simulink library "mylibrary"  (R2016b)
settings: Solver=VariableStepAuto  StartTime=0.0  StopTime=10.0  RelTol=1e-3
values from neighbouring files (symbols this model uses):
  bp_perio = bp_fft*2-3    (= 27)    [setup.m]
  Ewin = sum(wh.^2)/Nfft    [make_bias_plot_hann.m]    (also in setup.m = 1)
  N = M    [errAnalysis.m]    (also in make_bias_plot.m = 5; make_bias_plot_hann.m = 5; run_sim.m = 13; setup.m = 8)
  Nmax = 13    [setup.m]
  Ts = 1/fs    [create_test_vector.m]
libraries: xbsIndex_r4 x109, mylibrary x5, mylibrary_4printing x2
settings Model: Creator=susan  LastModifiedBy=292344
settings OptimizationCC: LifeSpan=inf
settings DebuggingCC: SFExecutionAtInitializationDiag=none

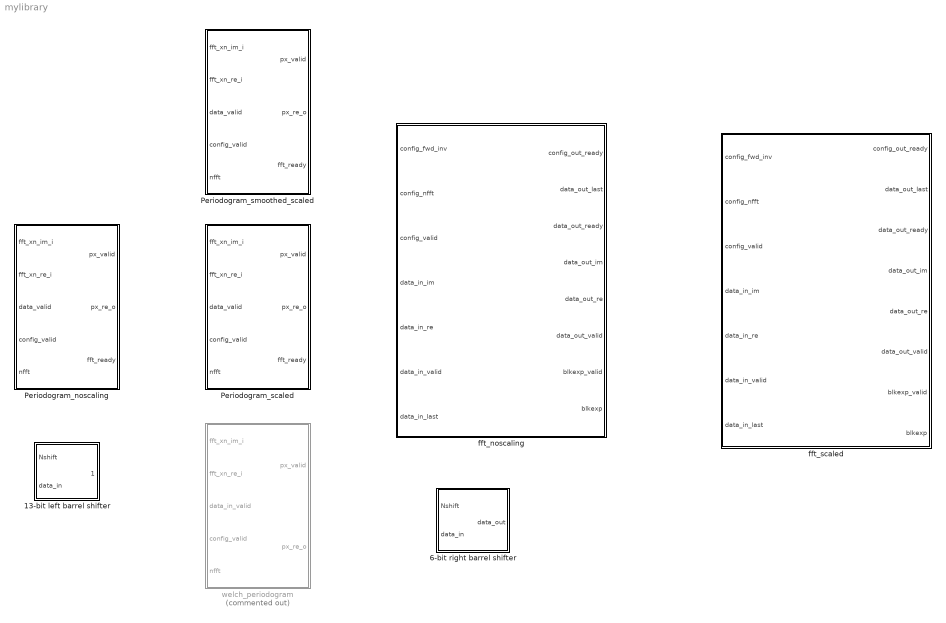
== system mylibrary ==
  13-bit left barrel shifter : Subsystem
  6-bit right barrel shifter : Subsystem
  Periodogram_noscaling : Subsystem
  Periodogram_scaled : Subsystem
  Periodogram_smoothed_scaled : Subsystem
  fft_noscaling : Subsystem
  fft_scaled : Subsystem
  welch_periodogram : Subsystem  Commented=on  AncestorBlock=mylibrary/smoothed_periodogram_scaled

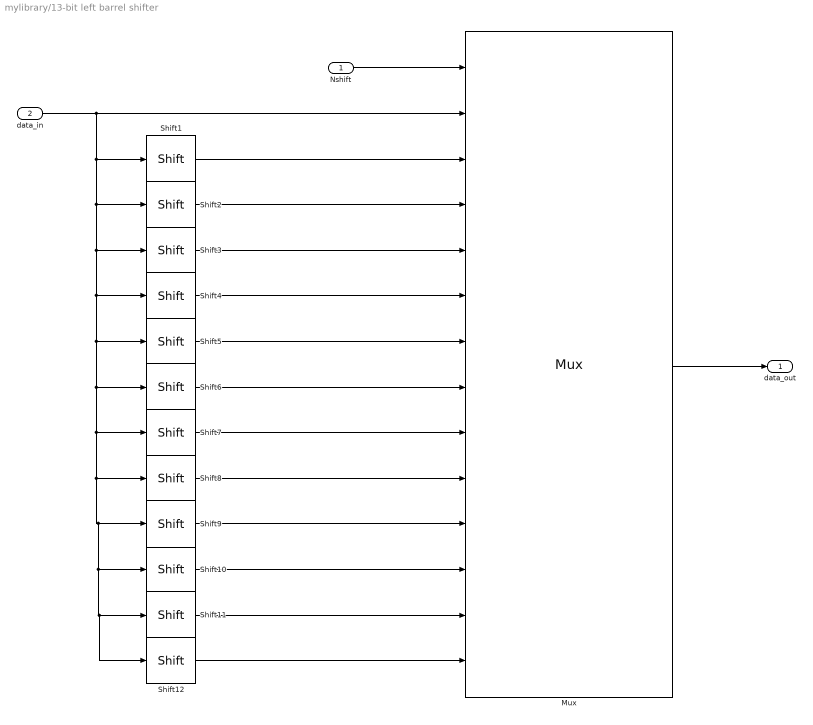
== system mylibrary/13-bit left barrel shifter ==
  Nshift : Inport
  data_in : Inport  Port=2
  Mux : xbsIndex_r4/Mux  inputs=13  en=off  latency=0  precision=Full  arith_type=Unsigned  n_bits=16  bin_pt=14  quantization=Truncate  overflow=Wrap  dbl_ovrd=off  block_type=mux
  Shift1 : xbsIndex_r4/Shift  shift_dir=Left  shift_bits=1  en=off  latency=0  precision=Full  arith_type="Signed  (2's comp)"  n_bits=16  bin_pt=14  quantization=Truncate  overflow=Wrap  dbl_ovrd=off  block_type=shift
  Shift10 : xbsIndex_r4/Shift  shift_dir=Left  shift_bits=10  en=off  latency=0  precision=Full  arith_type="Signed  (2's comp)"  n_bits=16  bin_pt=14  quantization=Truncate  overflow=Wrap  dbl_ovrd=off  block_type=shift
  Shift11 : xbsIndex_r4/Shift  shift_dir=Left  shift_bits=11  en=off  latency=0  precision=Full  arith_type="Signed  (2's comp)"  n_bits=16  bin_pt=14  quantization=Truncate  overflow=Wrap  dbl_ovrd=off  block_type=shift
  Shift12 : xbsIndex_r4/Shift  shift_dir=Left  shift_bits=12  en=off  latency=0  precision=Full  arith_type="Signed  (2's comp)"  n_bits=16  bin_pt=14  quantization=Truncate  overflow=Wrap  dbl_ovrd=off  block_type=shift
  Shift2 : xbsIndex_r4/Shift  shift_dir=Left  shift_bits=2  en=off  latency=0  precision=Full  arith_type="Signed  (2's comp)"  n_bits=16  bin_pt=14  quantization=Truncate  overflow=Wrap  dbl_ovrd=off  block_type=shift
  Shift3 : xbsIndex_r4/Shift  shift_dir=Left  shift_bits=3  en=off  latency=0  precision=Full  arith_type="Signed  (2's comp)"  n_bits=16  bin_pt=14  quantization=Truncate  overflow=Wrap  dbl_ovrd=off  block_type=shift
  Shift4 : xbsIndex_r4/Shift  shift_dir=Left  shift_bits=4  en=off  latency=0  precision=Full  arith_type="Signed  (2's comp)"  n_bits=16  bin_pt=14  quantization=Truncate  overflow=Wrap  dbl_ovrd=off  block_type=shift
  Shift5 : xbsIndex_r4/Shift  shift_dir=Left  shift_bits=5  en=off  latency=0  precision=Full  arith_type="Signed  (2's comp)"  n_bits=16  bin_pt=14  quantization=Truncate  overflow=Wrap  dbl_ovrd=off  block_type=shift
  Shift6 : xbsIndex_r4/Shift  shift_dir=Left  shift_bits=6  en=off  latency=0  precision=Full  arith_type="Signed  (2's comp)"  n_bits=16  bin_pt=14  quantization=Truncate  overflow=Wrap  dbl_ovrd=off  block_type=shift
  Shift7 : xbsIndex_r4/Shift  shift_dir=Left  shift_bits=7  en=off  latency=0  precision=Full  arith_type="Signed  (2's comp)"  n_bits=16  bin_pt=14  quantization=Truncate  overflow=Wrap  dbl_ovrd=off  block_type=shift
  Shift8 : xbsIndex_r4/Shift  shift_dir=Left  shift_bits=8  en=off  latency=0  precision=Full  arith_type="Signed  (2's comp)"  n_bits=16  bin_pt=14  quantization=Truncate  overflow=Wrap  dbl_ovrd=off  block_type=shift
  Shift9 : xbsIndex_r4/Shift  shift_dir=Left  shift_bits=9  en=off  latency=0  precision=Full  arith_type="Signed  (2's comp)"  n_bits=16  bin_pt=14  quantization=Truncate  overflow=Wrap  dbl_ovrd=off  block_type=shift
  data_out : Outport
  wires:
  Mux/1 -> data_out/1
  Nshift/1 -> Mux/1
  data_in/1 -> Shift12/1, Shift11/1, Shift10/1, Shift9/1, Shift8/1, Shift7/1, Shift6/1, Shift5/1, Shift4/1, Shift3/1, Shift2/1, Shift1/1, Mux/2
  Shift1/1 -> Mux/3
  Shift2/1 -> Mux/4
  Shift3/1 -> Mux/5
  Shift4/1 -> Mux/6
  Shift5/1 -> Mux/7
  Shift6/1 -> Mux/8
  Shift7/1 -> Mux/9
  Shift8/1 -> Mux/10
  Shift9/1 -> Mux/11
  Shift10/1 -> Mux/12
  Shift11/1 -> Mux/13
  Shift12/1 -> Mux/14

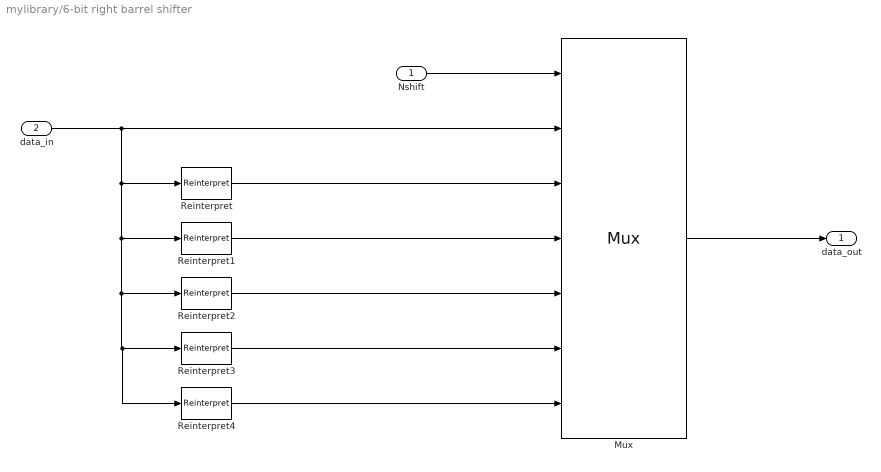
== system mylibrary/6-bit right barrel shifter ==
  Nshift : Inport
  data_in : Inport  Port=2
  Mux : xbsIndex_r4/Mux  inputs=6  en=off  latency=0  precision=Full  arith_type=Unsigned  n_bits=16  bin_pt=14  quantization=Truncate  overflow=Wrap  dbl_ovrd=off  block_type=mux
  Reinterpret : xbsIndex_r4/Reinterpret  force_arith_type=off  arith_type=Unsigned  force_bin_pt=on  bin_pt=bp_perio+1  block_type=reinterpret
  Reinterpret1 : xbsIndex_r4/Reinterpret  force_arith_type=off  arith_type=Unsigned  force_bin_pt=on  bin_pt=bp_perio+2  block_type=reinterpret
  Reinterpret2 : xbsIndex_r4/Reinterpret  force_arith_type=off  arith_type=Unsigned  force_bin_pt=on  bin_pt=bp_perio+3  block_type=reinterpret
  Reinterpret3 : xbsIndex_r4/Reinterpret  force_arith_type=off  arith_type=Unsigned  force_bin_pt=on  bin_pt=bp_perio+4  block_type=reinterpret
  Reinterpret4 : xbsIndex_r4/Reinterpret  force_arith_type=off  arith_type=Unsigned  force_bin_pt=on  bin_pt=bp_perio+5  block_type=reinterpret
  data_out : Outport
  wires:
  Nshift/1 -> Mux/1
  Mux/1 -> data_out/1
  Reinterpret/1 -> Mux/3
  Reinterpret1/1 -> Mux/4
  data_in/1 -> Reinterpret/1, Reinterpret4/1, Reinterpret3/1, Reinterpret2/1, Reinterpret1/1, Mux/2
  Reinterpret2/1 -> Mux/5
  Reinterpret3/1 -> Mux/6
  Reinterpret4/1 -> Mux/7

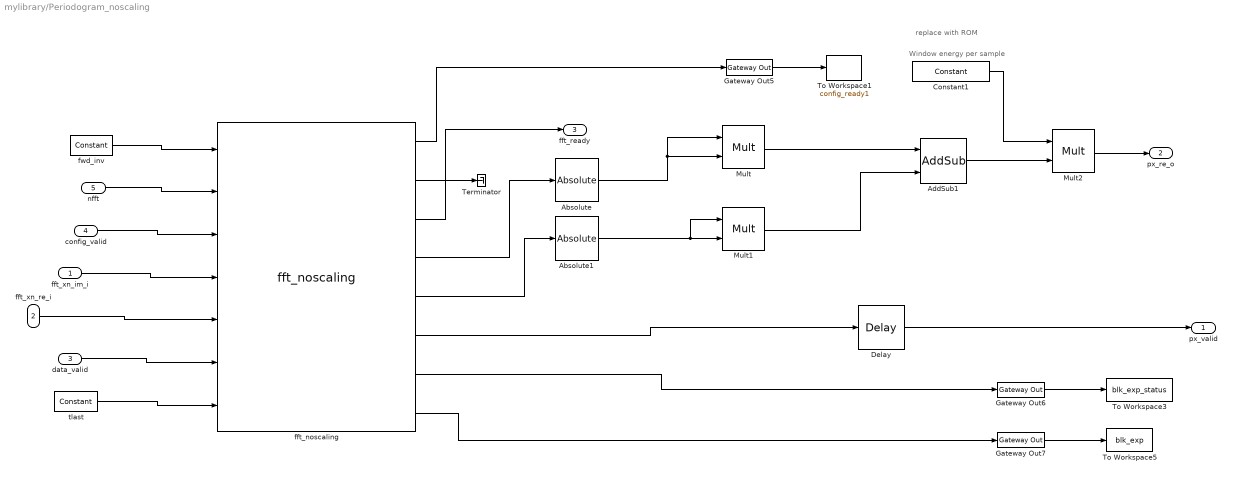
== system mylibrary/Periodogram_noscaling ==
  note: Window energy per sample
  note: replace with ROM
  fft_xn_im_i : Inport
  fft_xn_re_i : Inport  Port=2
  data_valid : Inport  Port=3
  config_valid : Inport  Port=4
  nfft : Inport  Port=5
  Absolute : xbsIndex_r4/Absolute  precision=User Defined  arith_type=Unsigned  n_bits=width_fft  bin_pt=bp_fft  quantization=Truncate  overflow=Wrap  en=off  latency=0  dbl_ovrd=off  block_type=abs
  Absolute1 : xbsIndex_r4/Absolute  precision=User Defined  arith_type=Unsigned  n_bits=width_fft  bin_pt=bp_fft  quantization=Truncate  overflow=Wrap  en=off  latency=0  dbl_ovrd=off  block_type=abs
  AddSub1 : xbsIndex_r4/AddSub  mode=Addition  use_carryin=off  use_carryout=off  en=off  latency=0  precision=Full  arith_type=Unsigned  n_bits=width_perio  bin_pt=bp_perio  quantization="Round  (unbiased: +/- Inf)"  overflow=Flag as error  use_behavioral_HDL=off  hw_selection=Fabric  pipelined=off  dbl_ovrd=off  block_type=addsub
  Constant1 : xbsIndex_r4/Constant  const=Ewin  gui_display_data_type=Fixed-point  arith_type=Unsigned  n_bits=32  bin_pt=20  preci_type=Single  exp_width=8  frac_width=24  explicit_period=on  period=1  equ=P=C  opselect=C  inp2=PCIN>>17  opr=+  inp1=P  carry=CIN  dbl_ovrd=off  block_type=constant
  Delay : xbsIndex_r4/Delay  rst=off  infoeditControl=Selection of Reset will increase slice count due to use of real FFs and instead of SRLs  en=off  latency=6  reg_retiming=off  dbl_ovrd=off  block_type=delay
      settings: infoedit=Hardware notes: A delay line is a chain, each link of which is an SRL16 or SRL32 followed by a flip-flop.
  Gateway Out5 : xbsIndex_r4/Gateway Out  inherit_from_input=off  hdl_port=on  rows=1  columns=1  UseAsDAC=off  DACChannel='1'  interface=None  automatic_assignment=on  address_offset=hex2dec('00')  intf_name=''  intf_description=''  timing_constraint=None  locs_specified=off  LOCs={}  io_standard={}  block_type=gatewayout
  Gateway Out6 : xbsIndex_r4/Gateway Out  inherit_from_input=off  hdl_port=on  rows=1  columns=1  UseAsDAC=off  DACChannel='1'  interface=None  automatic_assignment=on  address_offset=hex2dec('00')  intf_name=''  intf_description=''  timing_constraint=None  locs_specified=off  LOCs={}  io_standard={}  block_type=gatewayout
  Gateway Out7 : xbsIndex_r4/Gateway Out  inherit_from_input=off  hdl_port=on  rows=1  columns=1  UseAsDAC=off  DACChannel='1'  interface=None  automatic_assignment=on  address_offset=hex2dec('00')  intf_name=''  intf_description=''  timing_constraint=None  locs_specified=off  LOCs={}  io_standard={}  block_type=gatewayout
  Mult : xbsIndex_r4/Mult  precision=Full  arith_type=Unsigned  n_bits=width_perio  bin_pt=bp_perio  quantization="Round  (unbiased: +/- Inf)"  overflow=Wrap  en=off  latency=3  use_behavioral_HDL=off  opt=Speed  use_embedded=on  optimum_pipeline=off  pipeline=on  dbl_ovrd=off  use_rpm=on  placement_style=Triangular  block_type=mult
  Mult1 : xbsIndex_r4/Mult  precision=Full  arith_type=Unsigned  n_bits=width_perio  bin_pt=bp_perio  quantization="Round  (unbiased: +/- Inf)"  overflow=Wrap  en=off  latency=3  use_behavioral_HDL=off  opt=Speed  use_embedded=on  optimum_pipeline=off  pipeline=on  dbl_ovrd=off  use_rpm=on  placement_style=Triangular  block_type=mult
  Mult2 : xbsIndex_r4/Mult  precision=User Defined  arith_type=Unsigned  n_bits=width_perio  bin_pt=bp_perio  quantization="Round  (unbiased: +/- Inf)"  overflow=Flag as error  en=off  latency=3  use_behavioral_HDL=off  opt=Speed  use_embedded=on  optimum_pipeline=off  pipeline=on  dbl_ovrd=off  use_rpm=on  placement_style=Triangular  block_type=mult
  Terminator : Terminator
  To Workspace1 : ToWorkspace  VariableName=config_ready1  SaveFormat=Timeseries  SampleTime=-1
  To Workspace3 : ToWorkspace  VariableName=blk_exp_status  SaveFormat=Timeseries  SampleTime=-1
  To Workspace5 : ToWorkspace  VariableName=blk_exp  SaveFormat=Timeseries  SampleTime=-1
  fft_noscaling : mylibrary/fft_noscaling
  fwd_inv : xbsIndex_r4/Constant  const=1.0  gui_display_data_type=Fixed-point  arith_type=Unsigned  n_bits=1  bin_pt=0  preci_type=Single  exp_width=8  frac_width=24  explicit_period=off  period=1  equ=P=C  opselect=C  inp2=PCIN>>17  opr=+  inp1=P  carry=CIN  dbl_ovrd=off  block_type=constant
  tlast : xbsIndex_r4/Constant  const=1.0  gui_display_data_type=Boolean  arith_type=Boolean  n_bits=16  bin_pt=14  preci_type=Single  exp_width=8  frac_width=24  explicit_period=off  period=1  equ=P=C  opselect=C  inp2=PCIN>>17  opr=+  inp1=P  carry=CIN  dbl_ovrd=off  block_type=constant
  px_valid : Outport
  px_re_o : Outport  Port=2
  fft_ready : Outport  Port=3
  wires:
  Delay/1 -> px_valid/1
  Mult/1 -> AddSub1/1
  Mult1/1 -> AddSub1/2
  Gateway Out5/1 -> To Workspace1/1
  Absolute/1 -> Mult/2, Mult/1
  Absolute1/1 -> Mult1/1, Mult1/2
  AddSub1/1 -> Mult2/2
  Mult2/1 -> px_re_o/1
  Constant1/1 -> Mult2/1
  fft_noscaling/5 -> Absolute1/1
  fft_noscaling/6 -> Delay/1
  fft_noscaling/4 -> Absolute/1
  fwd_inv/1 -> fft_noscaling/1
  nfft/1 -> fft_noscaling/2
  config_valid/1 -> fft_noscaling/3
  fft_xn_im_i/1 -> fft_noscaling/4
  fft_xn_re_i/1 -> fft_noscaling/5
  data_valid/1 -> fft_noscaling/6
  tlast/1 -> fft_noscaling/7
  fft_noscaling/1 -> Gateway Out5/1
  fft_noscaling/3 -> fft_ready/1
  Gateway Out6/1 -> To Workspace3/1
  Gateway Out7/1 -> To Workspace5/1
  fft_noscaling/7 -> Gateway Out6/1
  fft_noscaling/8 -> Gateway Out7/1
  fft_noscaling/2 -> Terminator/1

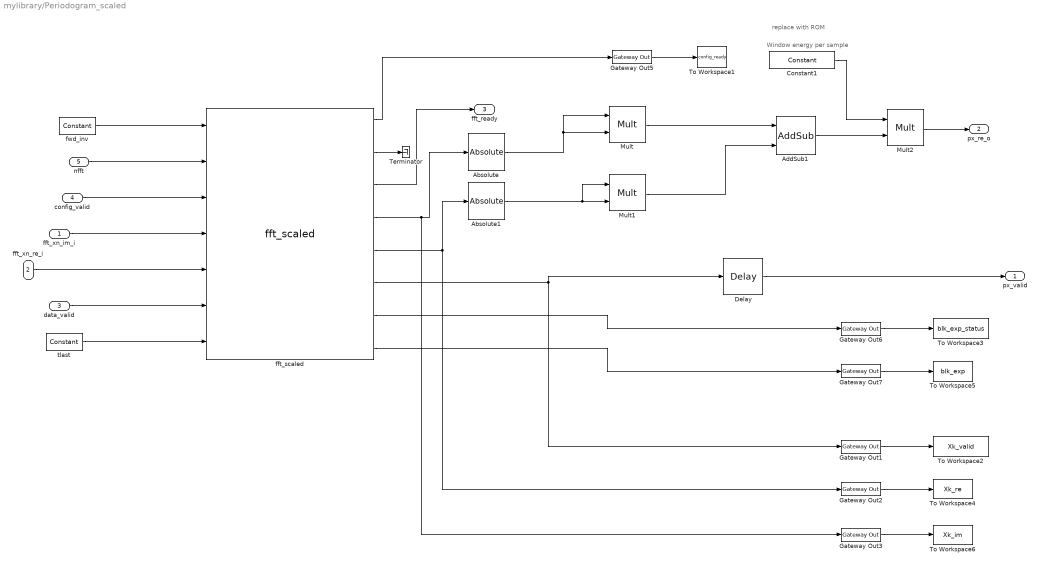
== system mylibrary/Periodogram_scaled ==
  note: replace with ROM
  note: Window energy per sample
  fft_xn_im_i : Inport
  fft_xn_re_i : Inport  Port=2
  data_valid : Inport  Port=3
  config_valid : Inport  Port=4
  nfft : Inport  Port=5
  Absolute : xbsIndex_r4/Absolute  precision=User Defined  arith_type=Unsigned  n_bits=width_fft  bin_pt=bp_fft  quantization=Truncate  overflow=Wrap  en=off  latency=0  dbl_ovrd=off  block_type=abs
  Absolute1 : xbsIndex_r4/Absolute  precision=User Defined  arith_type=Unsigned  n_bits=width_fft  bin_pt=bp_fft  quantization=Truncate  overflow=Wrap  en=off  latency=0  dbl_ovrd=off  block_type=abs
  AddSub1 : xbsIndex_r4/AddSub  mode=Addition  use_carryin=off  use_carryout=off  en=off  latency=0  precision=Full  arith_type=Unsigned  n_bits=width_perio  bin_pt=bp_perio  quantization="Round  (unbiased: +/- Inf)"  overflow=Flag as error  use_behavioral_HDL=off  hw_selection=Fabric  pipelined=off  dbl_ovrd=off  block_type=addsub
  Constant1 : xbsIndex_r4/Constant  const=Ewin  gui_display_data_type=Fixed-point  arith_type=Unsigned  n_bits=32  bin_pt=20  preci_type=Single  exp_width=8  frac_width=24  explicit_period=on  period=1  equ=P=C  opselect=C  inp2=PCIN>>17  opr=+  inp1=P  carry=CIN  dbl_ovrd=off  block_type=constant
  Delay : xbsIndex_r4/Delay  rst=off  infoeditControl=Selection of Reset will increase slice count due to use of real FFs and instead of SRLs  en=off  latency=6  reg_retiming=off  dbl_ovrd=off  block_type=delay
      settings: infoedit=Hardware notes: A delay line is a chain, each link of which is an SRL16 or SRL32 followed by a flip-flop.
  Gateway Out{1..3,5..7} (6 alike) : xbsIndex_r4/Gateway Out  inherit_from_input=off  hdl_port=on  rows=1  columns=1  UseAsDAC=off  DACChannel='1'  interface=None  automatic_assignment=on  address_offset=hex2dec('00')  intf_name=''  intf_description=''  timing_constraint=None  locs_specified=off  LOCs={}  io_standard={}  block_type=gatewayout
  Mult : xbsIndex_r4/Mult  precision=Full  arith_type=Unsigned  n_bits=width_perio  bin_pt=bp_perio  quantization="Round  (unbiased: +/- Inf)"  overflow=Wrap  en=off  latency=3  use_behavioral_HDL=off  opt=Speed  use_embedded=on  optimum_pipeline=off  pipeline=on  dbl_ovrd=off  use_rpm=on  placement_style=Triangular  block_type=mult
  Mult1 : xbsIndex_r4/Mult  precision=Full  arith_type=Unsigned  n_bits=width_perio  bin_pt=bp_perio  quantization="Round  (unbiased: +/- Inf)"  overflow=Wrap  en=off  latency=3  use_behavioral_HDL=off  opt=Speed  use_embedded=on  optimum_pipeline=off  pipeline=on  dbl_ovrd=off  use_rpm=on  placement_style=Triangular  block_type=mult
  Mult2 : xbsIndex_r4/Mult  precision=User Defined  arith_type=Unsigned  n_bits=width_perio  bin_pt=bp_perio  quantization="Round  (unbiased: +/- Inf)"  overflow=Flag as error  en=off  latency=3  use_behavioral_HDL=off  opt=Speed  use_embedded=on  optimum_pipeline=off  pipeline=on  dbl_ovrd=off  use_rpm=on  placement_style=Triangular  block_type=mult
  Terminator : Terminator
  To Workspace1 : ToWorkspace  VariableName=config_ready  SaveFormat=Timeseries  SampleTime=-1
  To Workspace2 : ToWorkspace  VariableName=Xk_valid  SaveFormat=Timeseries  SampleTime=-1
  To Workspace3 : ToWorkspace  VariableName=blk_exp_status  SaveFormat=Timeseries  SampleTime=-1
  To Workspace4 : ToWorkspace  VariableName=Xk_re  SaveFormat=Timeseries  SampleTime=-1
  To Workspace5 : ToWorkspace  VariableName=blk_exp  SaveFormat=Timeseries  SampleTime=-1
  To Workspace6 : ToWorkspace  VariableName=Xk_im  SaveFormat=Timeseries  SampleTime=-1
  fft_scaled : mylibrary/fft_scaled
  fwd_inv : xbsIndex_r4/Constant  const=1.0  gui_display_data_type=Fixed-point  arith_type=Unsigned  n_bits=1  bin_pt=0  preci_type=Single  exp_width=8  frac_width=24  explicit_period=off  period=1  equ=P=C  opselect=C  inp2=PCIN>>17  opr=+  inp1=P  carry=CIN  dbl_ovrd=off  block_type=constant
  tlast : xbsIndex_r4/Constant  const=1.0  gui_display_data_type=Boolean  arith_type=Boolean  n_bits=16  bin_pt=14  preci_type=Single  exp_width=8  frac_width=24  explicit_period=off  period=1  equ=P=C  opselect=C  inp2=PCIN>>17  opr=+  inp1=P  carry=CIN  dbl_ovrd=off  block_type=constant
  px_valid : Outport
  px_re_o : Outport  Port=2
  fft_ready : Outport  Port=3
  wires:
  fft_scaled/2 -> Terminator/1
  fft_scaled/8 -> Gateway Out7/1
  fft_scaled/7 -> Gateway Out6/1
  Gateway Out7/1 -> To Workspace5/1
  Gateway Out6/1 -> To Workspace3/1
  fft_scaled/3 -> fft_ready/1
  fft_scaled/1 -> Gateway Out5/1
  tlast/1 -> fft_scaled/7
  data_valid/1 -> fft_scaled/6
  fft_xn_re_i/1 -> fft_scaled/5
  fft_xn_im_i/1 -> fft_scaled/4
  config_valid/1 -> fft_scaled/3
  nfft/1 -> fft_scaled/2
  fwd_inv/1 -> fft_scaled/1
  fft_scaled/4 -> Gateway Out3/1, Absolute/1
  fft_scaled/6 -> Gateway Out1/1, Delay/1
  fft_scaled/5 -> Gateway Out2/1, Absolute1/1
  Constant1/1 -> Mult2/1
  Mult2/1 -> px_re_o/1
  AddSub1/1 -> Mult2/2
  Absolute1/1 -> Mult1/2, Mult1/1
  Absolute/1 -> Mult/1, Mult/2
  Gateway Out5/1 -> To Workspace1/1
  Mult1/1 -> AddSub1/2
  Mult/1 -> AddSub1/1
  Delay/1 -> px_valid/1
  Gateway Out2/1 -> To Workspace4/1
  Gateway Out1/1 -> To Workspace2/1
  Gateway Out3/1 -> To Workspace6/1

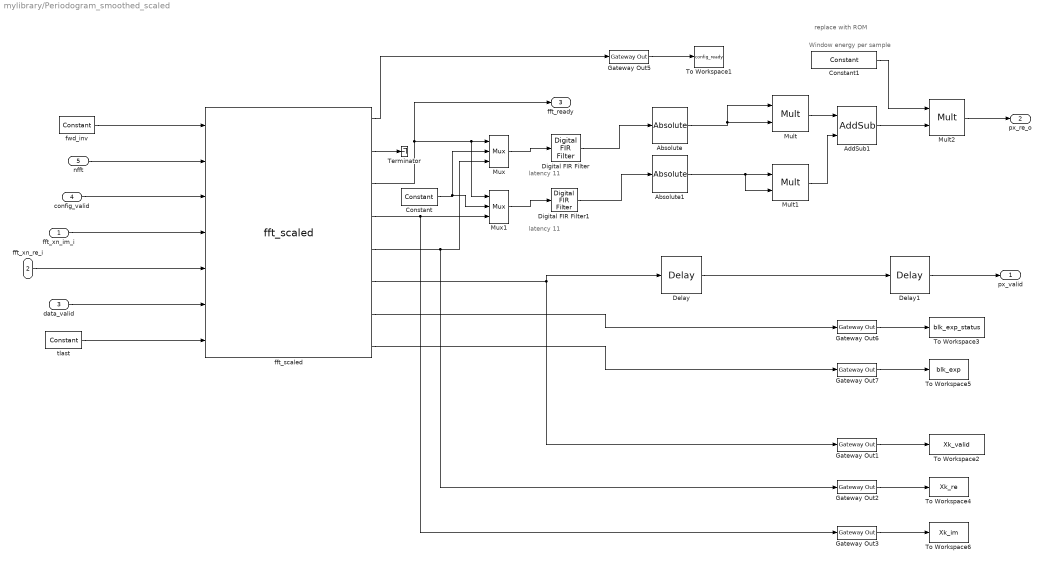
== system mylibrary/Periodogram_smoothed_scaled ==
  note: latency 11
  note: replace with ROM
  note: Window energy per sample
  note: latency 11
  fft_xn_im_i : Inport
  fft_xn_re_i : Inport  Port=2
  data_valid : Inport  Port=3
  config_valid : Inport  Port=4
  nfft : Inport  Port=5
  Absolute : xbsIndex_r4/Absolute  precision=User Defined  arith_type=Unsigned  n_bits=width_fft  bin_pt=bp_fft  quantization=Truncate  overflow=Wrap  en=off  latency=0  dbl_ovrd=off  block_type=abs
  Absolute1 : xbsIndex_r4/Absolute  precision=User Defined  arith_type=Unsigned  n_bits=width_fft  bin_pt=bp_fft  quantization=Truncate  overflow=Wrap  en=off  latency=0  dbl_ovrd=off  block_type=abs
  AddSub1 : xbsIndex_r4/AddSub  mode=Addition  use_carryin=off  use_carryout=off  en=off  latency=0  precision=Full  arith_type=Unsigned  n_bits=width_perio  bin_pt=bp_perio  quantization="Round  (unbiased: +/- Inf)"  overflow=Flag as error  use_behavioral_HDL=off  hw_selection=Fabric  pipelined=off  dbl_ovrd=off  block_type=addsub
  Constant : xbsIndex_r4/Constant  const=0  gui_display_data_type=Fixed-point  arith_type=Signed (2's comp)  n_bits=16  bin_pt=14  preci_type=Single  exp_width=8  frac_width=24  explicit_period=off  period=1  equ=P=C  opselect=C  inp2=PCIN>>17  opr=+  inp1=P  carry=CIN  dbl_ovrd=off  block_type=constant
  Constant1 : xbsIndex_r4/Constant  const=Ewin  gui_display_data_type=Fixed-point  arith_type=Unsigned  n_bits=32  bin_pt=20  preci_type=Single  exp_width=8  frac_width=24  explicit_period=on  period=1  equ=P=C  opselect=C  inp2=PCIN>>17  opr=+  inp1=P  carry=CIN  dbl_ovrd=off  block_type=constant
  Delay : xbsIndex_r4/Delay  rst=off  infoeditControl=Selection of Reset will increase slice count due to use of real FFs and instead of SRLs  en=off  latency=3  reg_retiming=off  dbl_ovrd=off  block_type=delay
  Delay1 : xbsIndex_r4/Delay  rst=off  infoeditControl=Selection of Reset will increase slice count due to use of real FFs and instead of SRLs  en=off  latency=14  reg_retiming=off  dbl_ovrd=off  block_type=delay
  Digital FIR Filter : xbsIndex_r4/Digital FIR Filter  coeff_source=off  coefficientvector=[-.25,0.5,-0.25]  coeff_calulate=on  coefficient_width=2  coefficient_fractional_bits=1  interpolation_filter_rate=1  decimation_filter_rate=1  fda_coefficientvector=[-0.0024 -0.0042 0.0095 0.0200 -0.0380 -0.0696 0.1374 0.4472 0.4472 0.1374 -0.0696 -0.0380 0.0200 0.0095 -0.0042 -0.0024]  simulation_type=fast_sim  simulation_model=sysgen:fir_macro  block_type=fir_macro
  Digital FIR Filter1 : xbsIndex_r4/Digital FIR Filter  coeff_source=off  coefficientvector=[-.25,0.5,-0.25]  coeff_calulate=on  coefficient_width=2  coefficient_fractional_bits=1  interpolation_filter_rate=1  decimation_filter_rate=1  fda_coefficientvector=[-0.0024 -0.0042 0.0095 0.0200 -0.0380 -0.0696 0.1374 0.4472 0.4472 0.1374 -0.0696 -0.0380 0.0200 0.0095 -0.0042 -0.0024]  simulation_type=fast_sim  simulation_model=sysgen:fir_macro  block_type=fir_macro
  Gateway Out{1..3,5..7} (6 alike) : xbsIndex_r4/Gateway Out  inherit_from_input=off  hdl_port=on  rows=1  columns=1  UseAsDAC=off  DACChannel='1'  interface=None  automatic_assignment=on  address_offset=hex2dec('00')  intf_name=''  intf_description=''  timing_constraint=None  locs_specified=off  LOCs={}  io_standard={}  block_type=gatewayout
  Mult : xbsIndex_r4/Mult  precision=Full  arith_type=Unsigned  n_bits=width_perio  bin_pt=bp_perio  quantization="Round  (unbiased: +/- Inf)"  overflow=Wrap  en=off  latency=3  use_behavioral_HDL=off  opt=Speed  use_embedded=on  optimum_pipeline=off  pipeline=on  dbl_ovrd=off  use_rpm=on  placement_style=Triangular  block_type=mult
  Mult1 : xbsIndex_r4/Mult  precision=Full  arith_type=Unsigned  n_bits=width_perio  bin_pt=bp_perio  quantization="Round  (unbiased: +/- Inf)"  overflow=Wrap  en=off  latency=3  use_behavioral_HDL=off  opt=Speed  use_embedded=on  optimum_pipeline=off  pipeline=on  dbl_ovrd=off  use_rpm=on  placement_style=Triangular  block_type=mult
  Mult2 : xbsIndex_r4/Mult  precision=User Defined  arith_type=Unsigned  n_bits=width_perio  bin_pt=bp_perio  quantization="Round  (unbiased: +/- Inf)"  overflow=Flag as error  en=off  latency=3  use_behavioral_HDL=off  opt=Speed  use_embedded=on  optimum_pipeline=off  pipeline=on  dbl_ovrd=off  use_rpm=on  placement_style=Triangular  block_type=mult
  Mux : xbsIndex_r4/Mux  inputs=2  en=off  latency=0  precision=Full  arith_type=Unsigned  n_bits=16  bin_pt=14  quantization=Truncate  overflow=Wrap  dbl_ovrd=off  block_type=mux
  Mux1 : xbsIndex_r4/Mux  inputs=2  en=off  latency=0  precision=Full  arith_type=Unsigned  n_bits=16  bin_pt=14  quantization=Truncate  overflow=Wrap  dbl_ovrd=off  block_type=mux
  Terminator : Terminator
  To Workspace1 : ToWorkspace  VariableName=config_ready  SaveFormat=Timeseries  SampleTime=-1
  To Workspace2 : ToWorkspace  VariableName=Xk_valid  SaveFormat=Timeseries  SampleTime=-1
  To Workspace3 : ToWorkspace  VariableName=blk_exp_status  SaveFormat=Timeseries  SampleTime=-1
  To Workspace4 : ToWorkspace  VariableName=Xk_re  SaveFormat=Timeseries  SampleTime=-1
  To Workspace5 : ToWorkspace  VariableName=blk_exp  SaveFormat=Timeseries  SampleTime=-1
  To Workspace6 : ToWorkspace  VariableName=Xk_im  SaveFormat=Timeseries  SampleTime=-1
  fft_scaled : mylibrary/fft_scaled
  fwd_inv : xbsIndex_r4/Constant  const=1.0  gui_display_data_type=Fixed-point  arith_type=Unsigned  n_bits=1  bin_pt=0  preci_type=Single  exp_width=8  frac_width=24  explicit_period=off  period=1  equ=P=C  opselect=C  inp2=PCIN>>17  opr=+  inp1=P  carry=CIN  dbl_ovrd=off  block_type=constant
  tlast : xbsIndex_r4/Constant  const=1.0  gui_display_data_type=Boolean  arith_type=Boolean  n_bits=16  bin_pt=14  preci_type=Single  exp_width=8  frac_width=24  explicit_period=off  period=1  equ=P=C  opselect=C  inp2=PCIN>>17  opr=+  inp1=P  carry=CIN  dbl_ovrd=off  block_type=constant
  px_valid : Outport
  px_re_o : Outport  Port=2
  fft_ready : Outport  Port=3
  wires:
  fft_scaled/2 -> Terminator/1
  fft_scaled/8 -> Gateway Out7/1
  fft_scaled/7 -> Gateway Out6/1
  Gateway Out7/1 -> To Workspace5/1
  Gateway Out6/1 -> To Workspace3/1
  fft_scaled/3 -> Mux1/1, Mux/1, fft_ready/1
  fft_scaled/1 -> Gateway Out5/1
  tlast/1 -> fft_scaled/7
  data_valid/1 -> fft_scaled/6
  fft_xn_re_i/1 -> fft_scaled/5
  fft_xn_im_i/1 -> fft_scaled/4
  config_valid/1 -> fft_scaled/3
  nfft/1 -> fft_scaled/2
  fwd_inv/1 -> fft_scaled/1
  fft_scaled/4 -> Mux1/3, Gateway Out3/1
  fft_scaled/6 -> Gateway Out1/1, Delay/1
  fft_scaled/5 -> Mux/3, Gateway Out2/1
  Constant1/1 -> Mult2/1
  Mult2/1 -> px_re_o/1
  Absolute1/1 -> Mult1/2, Mult1/1
  Absolute/1 -> Mult/1, Mult/2
  Gateway Out5/1 -> To Workspace1/1
  Mult1/1 -> AddSub1/2
  Mult/1 -> AddSub1/1
  Delay/1 -> Delay1/1
  Gateway Out2/1 -> To Workspace4/1
  Gateway Out1/1 -> To Workspace2/1
  Gateway Out3/1 -> To Workspace6/1
  Delay1/1 -> px_valid/1
  Mux/1 -> Digital FIR Filter/1
  AddSub1/1 -> Mult2/2
  Digital FIR Filter/1 -> Absolute/1
  Mux1/1 -> Digital FIR Filter1/1
  Digital FIR Filter1/1 -> Absolute1/1
  Constant/1 -> Mux1/2, Mux/2

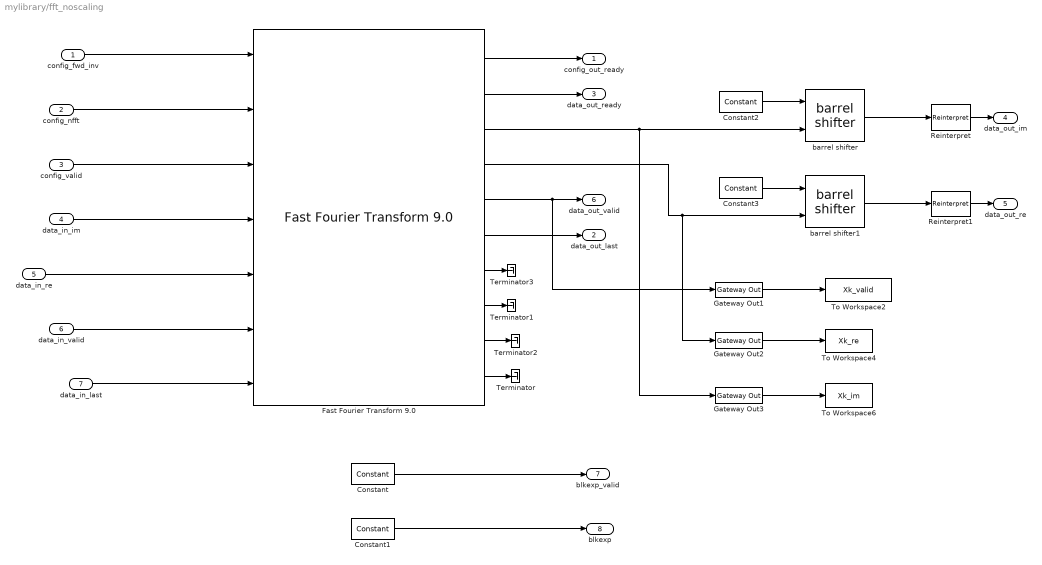
== system mylibrary/fft_noscaling ==
  config_fwd_inv : Inport
  config_nfft : Inport  Port=2
  config_valid : Inport  Port=3
  data_in_im : Inport  Port=4
  data_in_re : Inport  Port=5
  data_in_valid : Inport  Port=6
  data_in_last : Inport  Port=7
  Constant : xbsIndex_r4/Constant  const=1.0  gui_display_data_type=Boolean  arith_type=Boolean  n_bits=16  bin_pt=14  preci_type=Single  exp_width=8  frac_width=24  explicit_period=off  period=1  equ=P=C  opselect=C  inp2=PCIN>>17  opr=+  inp1=P  carry=CIN  dbl_ovrd=off  block_type=constant
  Constant1 : xbsIndex_r4/Constant  const=N  gui_display_data_type=Fixed-point  arith_type=Unsigned  n_bits=5  bin_pt=0  preci_type=Single  exp_width=8  frac_width=24  explicit_period=off  period=1  equ=P=C  opselect=C  inp2=PCIN>>17  opr=+  inp1=P  carry=CIN  dbl_ovrd=off  block_type=constant
  Constant2 : xbsIndex_r4/Constant  const=Nmax-N  gui_display_data_type=Fixed-point  arith_type=Unsigned  n_bits=4  bin_pt=0  preci_type=Single  exp_width=8  frac_width=24  explicit_period=off  period=1  equ=P=C  opselect=C  inp2=PCIN>>17  opr=+  inp1=P  carry=CIN  dbl_ovrd=off  block_type=constant
  Constant3 : xbsIndex_r4/Constant  const=Nmax-N  gui_display_data_type=Fixed-point  arith_type=Unsigned  n_bits=4  bin_pt=0  preci_type=Single  exp_width=8  frac_width=24  explicit_period=off  period=1  equ=P=C  opselect=C  inp2=PCIN>>17  opr=+  inp1=P  carry=CIN  dbl_ovrd=off  block_type=constant
  "Fast Fourier Transform 9.0 " : xbsIndex_r4/Fast Fourier Transform 9.0   transform_length=8192  target_clock_frequency=ceil(1/(Ts*1e6))  target_data_throughput=50  implementation_options=pipelined_streaming_io  run_time_configurable_transform_length=on  phase_factor_width=13  scaling_options=unscaled  rounding_modes=convergent_rounding  aclken=off  aresetn=off  output_ordering=natural_order  cyclic_prefix_insertion=off  throttle_scheme=realtime  xk_index=off  ovflo=off  trim_axipin_name=on  memory_options_data=block_ram  memory_options_phase_factors=block_ram  number_of_stages_using_block_ram_for_data_and_phase_factors=4  memory_options_reorder=block_ram  memory_options_hybrid=off  complex_mult_type=use_mults_performance  butterfly_type=use_luts  simulation_type=hybrid_sim  simulation_model=sysgen:xfftv9_cmodel  data_path_portlist={ 's_axis_data_tdata', 'm_axis_data_tdata', 'm_axis_status_tdata', 'event_fft_overflow' }  channels=1  input_ordering=natural_order  input_width=16  ip_name=Fast Fourier Transform  ip_version=9.0  dsptool_ready=true  ipcore_usecache=true  ipcore_useipmodelcache=true  wrapper_available=true  port_translation_map={ 'aclken' => 'en', 'aresetn' => 'rst'}  data_format=fixed_point  block_type=xfft_v9_0
  Gateway Out1 : xbsIndex_r4/Gateway Out  inherit_from_input=off  hdl_port=on  rows=1  columns=1  UseAsDAC=off  DACChannel='1'  interface=None  automatic_assignment=on  address_offset=hex2dec('00')  intf_name=''  intf_description=''  timing_constraint=None  locs_specified=off  LOCs={}  io_standard={}  block_type=gatewayout
  Gateway Out2 : xbsIndex_r4/Gateway Out  inherit_from_input=off  hdl_port=on  rows=1  columns=1  UseAsDAC=off  DACChannel='1'  interface=None  automatic_assignment=on  address_offset=hex2dec('00')  intf_name=''  intf_description=''  timing_constraint=None  locs_specified=off  LOCs={}  io_standard={}  block_type=gatewayout
  Gateway Out3 : xbsIndex_r4/Gateway Out  inherit_from_input=off  hdl_port=on  rows=1  columns=1  UseAsDAC=off  DACChannel='1'  interface=None  automatic_assignment=on  address_offset=hex2dec('00')  intf_name=''  intf_description=''  timing_constraint=None  locs_specified=off  LOCs={}  io_standard={}  block_type=gatewayout
  Reinterpret : xbsIndex_r4/Reinterpret  force_arith_type=off  arith_type=Unsigned  force_bin_pt=on  bin_pt=bp_reinterp  block_type=reinterpret
  Reinterpret1 : xbsIndex_r4/Reinterpret  force_arith_type=off  arith_type=Unsigned  force_bin_pt=on  bin_pt=bp_reinterp  block_type=reinterpret
  Terminator{,1..3} (4 alike) : Terminator
  To Workspace2 : ToWorkspace  VariableName=Xk_valid  SaveFormat=Timeseries  SampleTime=-1
  To Workspace4 : ToWorkspace  VariableName=Xk_re  SaveFormat=Timeseries  SampleTime=-1
  To Workspace6 : ToWorkspace  VariableName=Xk_im  SaveFormat=Timeseries  SampleTime=-1
  barrel shifter : mylibrary_4printing/barrel shifter
  barrel shifter1 : mylibrary_4printing/barrel shifter
  config_out_ready : Outport
  data_out_last : Outport  Port=2
  data_out_ready : Outport  Port=3
  data_out_im : Outport  Port=4
  data_out_re : Outport  Port=5
  data_out_valid : Outport  Port=6
  blkexp_valid : Outport  Port=7
  blkexp : Outport  Port=8
  wires:
  config_fwd_inv/1 -> "Fast Fourier Transform 9.0 "/1
  "Fast Fourier Transform 9.0 "/2 -> data_out_ready/1
  "Fast Fourier Transform 9.0 "/1 -> config_out_ready/1
  config_nfft/1 -> "Fast Fourier Transform 9.0 "/2
  data_in_im/1 -> "Fast Fourier Transform 9.0 "/4
  data_in_re/1 -> "Fast Fourier Transform 9.0 "/5
  data_in_last/1 -> "Fast Fourier Transform 9.0 "/7
  data_in_valid/1 -> "Fast Fourier Transform 9.0 "/6
  config_valid/1 -> "Fast Fourier Transform 9.0 "/3
  "Fast Fourier Transform 9.0 "/10 -> Terminator/1
  "Fast Fourier Transform 9.0 "/8 -> Terminator1/1
  "Fast Fourier Transform 9.0 "/9 -> Terminator2/1
  "Fast Fourier Transform 9.0 "/7 -> Terminator3/1
  Constant/1 -> blkexp_valid/1
  Constant1/1 -> blkexp/1
  "Fast Fourier Transform 9.0 "/5 -> Gateway Out1/1, data_out_valid/1
  "Fast Fourier Transform 9.0 "/6 -> data_out_last/1
  "Fast Fourier Transform 9.0 "/3 -> Gateway Out3/1, barrel shifter/2
  "Fast Fourier Transform 9.0 "/4 -> Gateway Out2/1, barrel shifter1/2
  barrel shifter/1 -> Reinterpret/1
  Reinterpret/1 -> data_out_im/1
  Reinterpret1/1 -> data_out_re/1
  Constant2/1 -> barrel shifter/1
  Constant3/1 -> barrel shifter1/1
  barrel shifter1/1 -> Reinterpret1/1
  Gateway Out3/1 -> To Workspace6/1
  Gateway Out1/1 -> To Workspace2/1
  Gateway Out2/1 -> To Workspace4/1

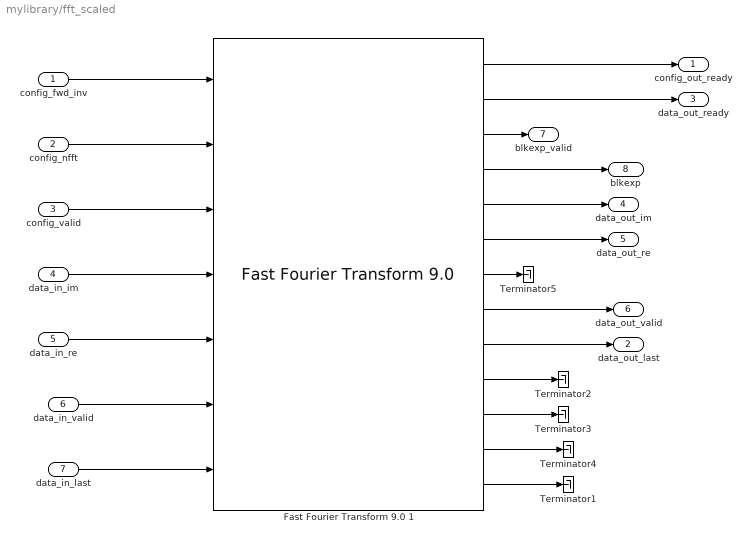
== system mylibrary/fft_scaled ==
  config_fwd_inv : Inport
  config_nfft : Inport  Port=2
  config_valid : Inport  Port=3
  data_in_im : Inport  Port=4
  data_in_re : Inport  Port=5
  data_in_valid : Inport  Port=6
  data_in_last : Inport  Port=7
  Fast Fourier Transform 9.0 1 : xbsIndex_r4/Fast Fourier Transform 9.0   transform_length=8192  target_clock_frequency=ceil(1/(Ts*1e6))  target_data_throughput=50  implementation_options=pipelined_streaming_io  run_time_configurable_transform_length=on  phase_factor_width=13  scaling_options=block_floating_point  rounding_modes=convergent_rounding  aclken=off  aresetn=off  output_ordering=natural_order  cyclic_prefix_insertion=off  throttle_scheme=realtime  xk_index=off  ovflo=off  trim_axipin_name=on  memory_options_data=block_ram  memory_options_phase_factors=block_ram  number_of_stages_using_block_ram_for_data_and_phase_factors=4  memory_options_reorder=block_ram  memory_options_hybrid=off  complex_mult_type=use_mults_performance  butterfly_type=use_luts  simulation_type=hybrid_sim  simulation_model=sysgen:xfftv9_cmodel  data_path_portlist={ 's_axis_data_tdata', 'm_axis_data_tdata', 'm_axis_status_tdata', 'event_fft_overflow' }  channels=1  input_ordering=natural_order  input_width=16  ip_name=Fast Fourier Transform  ip_version=9.0  dsptool_ready=true  ipcore_usecache=true  ipcore_useipmodelcache=true  wrapper_available=true  port_translation_map={ 'aclken' => 'en', 'aresetn' => 'rst'}  data_format=fixed_point  block_type=xfft_v9_0
  Terminator{1..5} (5 alike) : Terminator
  config_out_ready : Outport
  data_out_last : Outport  Port=2
  data_out_ready : Outport  Port=3
  data_out_im : Outport  Port=4
  data_out_re : Outport  Port=5
  data_out_valid : Outport  Port=6
  blkexp_valid : Outport  Port=7
  blkexp : Outport  Port=8
  wires:
  config_fwd_inv/1 -> Fast Fourier Transform 9.0 1/1
  config_nfft/1 -> Fast Fourier Transform 9.0 1/2
  data_in_im/1 -> Fast Fourier Transform 9.0 1/4
  data_in_last/1 -> Fast Fourier Transform 9.0 1/7
  data_in_valid/1 -> Fast Fourier Transform 9.0 1/6
  config_valid/1 -> Fast Fourier Transform 9.0 1/3
  Fast Fourier Transform 9.0 1/3 -> blkexp_valid/1
  data_in_re/1 -> Fast Fourier Transform 9.0 1/5
  Fast Fourier Transform 9.0 1/2 -> data_out_ready/1
  Fast Fourier Transform 9.0 1/9 -> data_out_last/1
  Fast Fourier Transform 9.0 1/1 -> config_out_ready/1
  Fast Fourier Transform 9.0 1/5 -> data_out_im/1
  Fast Fourier Transform 9.0 1/6 -> data_out_re/1
  Fast Fourier Transform 9.0 1/8 -> data_out_valid/1
  Fast Fourier Transform 9.0 1/13 -> Terminator1/1
  Fast Fourier Transform 9.0 1/10 -> Terminator2/1
  Fast Fourier Transform 9.0 1/11 -> Terminator3/1
  Fast Fourier Transform 9.0 1/12 -> Terminator4/1
  Fast Fourier Transform 9.0 1/4 -> blkexp/1
  Fast Fourier Transform 9.0 1/7 -> Terminator5/1

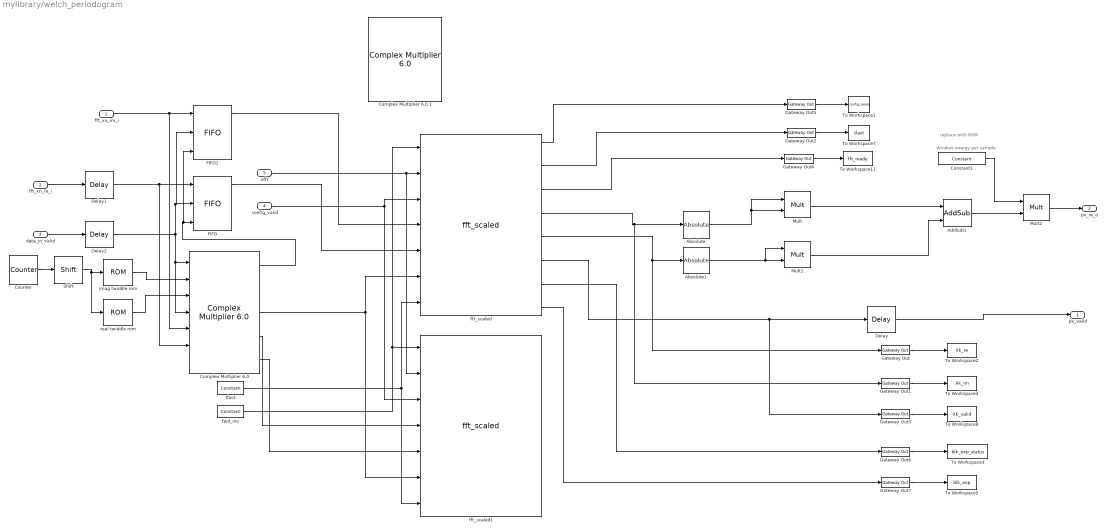
== system mylibrary/welch_periodogram ==
  note: Window energy per sample
  note: replace with ROM
  fft_xn_im_i : Inport
  fft_xn_re_i : Inport  Port=2
  data_in_valid : Inport  Port=3
  config_valid : Inport  Port=4
  nfft : Inport  Port=5
  Absolute : xbsIndex_r4/Absolute  precision=User Defined  arith_type=Unsigned  n_bits=width_fft  bin_pt=bp_fft  quantization=Truncate  overflow=Wrap  en=off  latency=0  dbl_ovrd=off  block_type=abs
  Absolute1 : xbsIndex_r4/Absolute  precision=User Defined  arith_type=Unsigned  n_bits=width_fft  bin_pt=bp_fft  quantization=Truncate  overflow=Wrap  en=off  latency=0  dbl_ovrd=off  block_type=abs
  AddSub1 : xbsIndex_r4/AddSub  mode=Addition  use_carryin=off  use_carryout=off  en=off  latency=0  precision=Full  arith_type=Unsigned  n_bits=width_perio  bin_pt=bp_perio  quantization="Round  (unbiased: +/- Inf)"  overflow=Flag as error  use_behavioral_HDL=off  hw_selection=Fabric  pipelined=off  dbl_ovrd=off  block_type=addsub
  "Complex Multiplier 6.0 " : xbsIndex_r4/Complex Multiplier 6.0   hasatlast=off  hasatuser=off  atuserwidth=1  hasbtlast=off  hasbtuser=off  btuserwidth=1  multtype=Use_Mults  optimizegoal=Resources  flowcontrol=Blocking  outputwidth=16  roundmode=Truncate  hasctrltlast=off  hasctrltuser=off  ctrltuserwidth=1  outtlastbehv=Null  latencyconfig=Automatic  minimumlatency=40  aclken=off  aresetn=off  trim_axipin_name=on  simulation_type=hybrid_sim  simulation_model=sysgen:cmpy_v6_0  data_path_portlist={ 's_axis_a_tdata_real', 's_axis_a_tdata_imag', 's_axis_b_tdata_real', 's_axis_b_tdata_imag', 's_axis_ctrl_tdata_rounding_bit', 'm_axis_dout_tdata_real', 'm_axis_dout_tdata_imag' }  aportwidth=63  bportwidth=63  ip_name=Complex Multiplier  ip_version=6.0  dsptool_ready=true  ipcore_usecache=true  ipcore_useipmodelcache=true  ipcore_verbose=false  ipcore_latency_parameter='minimumlatency'  wrapper_available=true  port_translation_map={ 'aclken' => 'en', 'aresetn' => 'rst'}  block_type=cmpy_v6_0
  Complex Multiplier 6.0 1 : xbsIndex_r4/Complex Multiplier 6.0   hasatlast=off  hasatuser=off  atuserwidth=1  hasbtlast=off  hasbtuser=off  btuserwidth=1  multtype=Use_Mults  optimizegoal=Resources  flowcontrol=NonBlocking  outputwidth=33  roundmode=Truncate  hasctrltlast=off  hasctrltuser=off  ctrltuserwidth=1  outtlastbehv=Null  latencyconfig=Automatic  minimumlatency=15  aclken=off  aresetn=off  trim_axipin_name=on  simulation_type=hybrid_sim  simulation_model=sysgen:cmpy_v6_0  data_path_portlist={ 's_axis_a_tdata_real', 's_axis_a_tdata_imag', 's_axis_b_tdata_real', 's_axis_b_tdata_imag', 's_axis_ctrl_tdata_rounding_bit', 'm_axis_dout_tdata_real', 'm_axis_dout_tdata_imag' }  aportwidth=63  bportwidth=63  ip_name=Complex Multiplier  ip_version=6.0  dsptool_ready=true  ipcore_usecache=true  ipcore_useipmodelcache=true  ipcore_verbose=false  ipcore_latency_parameter='minimumlatency'  wrapper_available=true  port_translation_map={ 'aclken' => 'en', 'aresetn' => 'rst'}  block_type=cmpy_v6_0
  Constant1 : xbsIndex_r4/Constant  const=Ewin  gui_display_data_type=Fixed-point  arith_type=Unsigned  n_bits=16  bin_pt=15  preci_type=Single  exp_width=8  frac_width=24  explicit_period=on  period=1  equ=P=C  opselect=C  inp2=PCIN>>17  opr=+  inp1=P  carry=CIN  dbl_ovrd=off  block_type=constant
  Counter : xbsIndex_r4/Counter  cnt_type=Free Running  cnt_to=Inf  operation=Up  start_count=0  cnt_by_val=1  arith_type=Unsigned  n_bits=Nmax  bin_pt=0  load_pin=off  rst=off  en=off  explicit_period=on  period=1  use_behavioral_HDL=off  implementation=Fabric  dbl_ovrd=off  block_type=counter
  Delay : xbsIndex_r4/Delay  rst=off  infoeditControl=Selection of Reset will increase slice count due to use of real FFs and instead of SRLs  en=off  latency=6  reg_retiming=off  dbl_ovrd=off  block_type=delay
      settings: infoedit=Hardware notes: A delay line is a chain, each link of which is an SRL16 or SRL32 followed by a flip-flop.
  Delay1 : xbsIndex_r4/Delay  rst=off  infoeditControl=Selection of Reset will increase slice count due to use of real FFs and instead of SRLs  en=off  latency=2  reg_retiming=off  dbl_ovrd=off  block_type=delay
  Delay2 : xbsIndex_r4/Delay  rst=off  infoeditControl=Selection of Reset will increase slice count due to use of real FFs and instead of SRLs  en=off  latency=2  reg_retiming=off  dbl_ovrd=off  block_type=delay
  FIFO : xbsIndex_r4/FIFO  mem_type=Block RAM  performance_options=Standard_FIFO  embedded_registers=off  depth=16  percent_nbits=1  rst=off  rst_latency=1  en=off  use_dcount=off  use_percent_full_port=off  use_almost_empty=off  almost_empty_thresh=2  use_almost_full=off  almost_full_thresh=14  explicit_period=off  dbl_ovrd=off  block_type=fifo
  FIFO1 : xbsIndex_r4/FIFO  mem_type=Block RAM  performance_options=Standard_FIFO  embedded_registers=off  depth=16  percent_nbits=1  rst=off  rst_latency=1  en=off  use_dcount=off  use_percent_full_port=off  use_almost_empty=off  almost_empty_thresh=2  use_almost_full=off  almost_full_thresh=14  explicit_period=off  dbl_ovrd=off  block_type=fifo
  Gateway Out{,1..7} (8 alike) : xbsIndex_r4/Gateway Out  inherit_from_input=off  hdl_port=on  rows=1  columns=1  UseAsDAC=off  DACChannel='1'  interface=None  automatic_assignment=on  address_offset=hex2dec('00')  intf_name=''  intf_description=''  timing_constraint=None  locs_specified=off  LOCs={}  io_standard={}  block_type=gatewayout
  Mult : xbsIndex_r4/Mult  precision=Full  arith_type=Unsigned  n_bits=width_perio  bin_pt=bp_perio  quantization="Round  (unbiased: +/- Inf)"  overflow=Wrap  en=off  latency=3  use_behavioral_HDL=off  opt=Speed  use_embedded=on  optimum_pipeline=off  pipeline=on  dbl_ovrd=off  use_rpm=on  placement_style=Triangular  block_type=mult
  Mult1 : xbsIndex_r4/Mult  precision=Full  arith_type=Unsigned  n_bits=width_perio  bin_pt=bp_perio  quantization="Round  (unbiased: +/- Inf)"  overflow=Wrap  en=off  latency=3  use_behavioral_HDL=off  opt=Speed  use_embedded=on  optimum_pipeline=off  pipeline=on  dbl_ovrd=off  use_rpm=on  placement_style=Triangular  block_type=mult
  Mult2 : xbsIndex_r4/Mult  precision=User Defined  arith_type=Unsigned  n_bits=width_perio  bin_pt=bp_perio  quantization="Round  (unbiased: +/- Inf)"  overflow=Flag as error  en=off  latency=3  use_behavioral_HDL=off  opt=Speed  use_embedded=on  optimum_pipeline=off  pipeline=on  dbl_ovrd=off  use_rpm=on  placement_style=Triangular  block_type=mult
  Shift : xbsIndex_r4/Shift  shift_dir=Left  shift_bits=Nmax-N  en=off  latency=0  precision=Full  arith_type="Signed  (2's comp)"  n_bits=16  bin_pt=14  quantization=Truncate  overflow=Wrap  dbl_ovrd=off  block_type=shift
  To Workspace1 : ToWorkspace  VariableName=config_ready  SaveFormat=Timeseries  SampleTime=-1
  To Workspace11 : ToWorkspace  VariableName=fft_ready  SaveFormat=Timeseries  SampleTime=-1
  To Workspace2 : ToWorkspace  VariableName=Xk_re  SaveFormat=Timeseries  SampleTime=-1
  To Workspace3 : ToWorkspace  VariableName=blk_exp_status  SaveFormat=Timeseries  SampleTime=-1
  To Workspace4 : ToWorkspace  VariableName=Xk_im  SaveFormat=Timeseries  SampleTime=-1
  To Workspace5 : ToWorkspace  VariableName=blk_exp  SaveFormat=Timeseries  SampleTime=-1
  To Workspace7 : ToWorkspace  VariableName=tlast  SaveFormat=Timeseries  SampleTime=-1
  To Workspace8 : ToWorkspace  VariableName=Xk_valid  SaveFormat=Timeseries  SampleTime=-1
  fft_scaled : mylibrary/fft_scaled
  fft_scaled1 : mylibrary/fft_scaled
  fwd_inv : xbsIndex_r4/Constant  const=1.0  gui_display_data_type=Fixed-point  arith_type=Unsigned  n_bits=1  bin_pt=0  preci_type=Single  exp_width=8  frac_width=24  explicit_period=off  period=1  equ=P=C  opselect=C  inp2=PCIN>>17  opr=+  inp1=P  carry=CIN  dbl_ovrd=off  block_type=constant
  imag twiddle rom : xbsIndex_r4/ROM  depth=16  initVector=imagtwiddles  distributed_mem=Block RAM  rst=off  init_reg=0  en=off  latency=1  gui_display_data_type=Fixed-point  arith_type="Signed  (2's comp)"  n_bits=16  bin_pt=14  preci_type=Single  exp_width=8  frac_width=24  optimize=Area  use_rpm=on  dbl_ovrd=off  block_type=sprom
  real twiddle rom : xbsIndex_r4/ROM  depth=16  initVector=realtwiddles  distributed_mem=Block RAM  rst=off  init_reg=0  en=off  latency=1  gui_display_data_type=Fixed-point  arith_type="Signed  (2's comp)"  n_bits=16  bin_pt=14  preci_type=Single  exp_width=8  frac_width=24  optimize=Area  use_rpm=on  dbl_ovrd=off  block_type=sprom
  tlast : xbsIndex_r4/Constant  const=1.0  gui_display_data_type=Boolean  arith_type=Boolean  n_bits=16  bin_pt=14  preci_type=Single  exp_width=8  frac_width=24  explicit_period=off  period=1  equ=P=C  opselect=C  inp2=PCIN>>17  opr=+  inp1=P  carry=CIN  dbl_ovrd=off  block_type=constant
  px_valid : Outport
  px_re_o : Outport  Port=2
  wires:
  Delay/1 -> px_valid/1
  Mult/1 -> AddSub1/1
  Mult1/1 -> AddSub1/2
  Gateway Out4/1 -> To Workspace11/1
  Gateway Out1/1 -> To Workspace4/1
  Gateway Out/1 -> To Workspace2/1
  Gateway Out2/1 -> To Workspace7/1
  Gateway Out3/1 -> To Workspace8/1
  Gateway Out5/1 -> To Workspace1/1
  Absolute/1 -> Mult/2, Mult/1
  Absolute1/1 -> Mult1/1, Mult1/2
  AddSub1/1 -> Mult2/2
  Mult2/1 -> px_re_o/1
  Constant1/1 -> Mult2/1
  fft_scaled/1 -> Gateway Out5/1
  fft_scaled/2 -> Gateway Out2/1
  fft_scaled/3 -> Gateway Out4/1
  Gateway Out6/1 -> To Workspace3/1
  Gateway Out7/1 -> To Workspace5/1
  fft_scaled/7 -> Gateway Out6/1
  fft_scaled/8 -> Gateway Out7/1
  fft_scaled/6 -> Gateway Out3/1, Delay/1
  fft_scaled/5 -> Gateway Out/1, Absolute1/1
  fft_scaled/4 -> Gateway Out1/1, Absolute/1
  imag twiddle rom/1 -> "Complex Multiplier 6.0 "/2
  real twiddle rom/1 -> "Complex Multiplier 6.0 "/3
  fwd_inv/1 -> fft_scaled/1, fft_scaled1/1
  tlast/1 -> fft_scaled1/7, fft_scaled/7
  FIFO1/1 -> fft_scaled/4
  FIFO/1 -> fft_scaled/5
  "Complex Multiplier 6.0 "/1 -> FIFO1/3, FIFO/3
  fft_xn_im_i/1 -> FIFO1/1, "Complex Multiplier 6.0 "/5
  fft_xn_re_i/1 -> Delay1/1
  Shift/1 -> real twiddle rom/1, imag twiddle rom/1
  Counter/1 -> Shift/1
  data_in_valid/1 -> Delay2/1
  nfft/1 -> fft_scaled1/2, fft_scaled/2
  config_valid/1 -> fft_scaled/3, fft_scaled1/3
  "Complex Multiplier 6.0 "/3 -> fft_scaled1/6, fft_scaled/6
  "Complex Multiplier 6.0 "/5 -> fft_scaled1/5
  "Complex Multiplier 6.0 "/4 -> fft_scaled1/4
  Delay1/1 -> "Complex Multiplier 6.0 "/6, FIFO/1
  Delay2/1 -> "Complex Multiplier 6.0 "/4, "Complex Multiplier 6.0 "/1, FIFO1/2, FIFO/2
